simulink model "example_3_cascaded_attitude"  (R2016a)
settings: Solver=VariableStepAuto  StartTime=0.0  StopTime=Tsim  MaxStep=0.01  RelTol=1e-3
values from neighbouring files (symbols this model uses):
  ref_A = [4, 4, 4]    [init.m]
  ref_b = [0, 0, 0]    [init.m]
  ref_p = [1, 2, 3]    [init.m]
  ref_w = [0,0,0]    [init.m]
libraries: aerolibtransform2 x5, vrlib x3
settings Model: Creator=mgreiff  LastModifiedBy=mgreiff

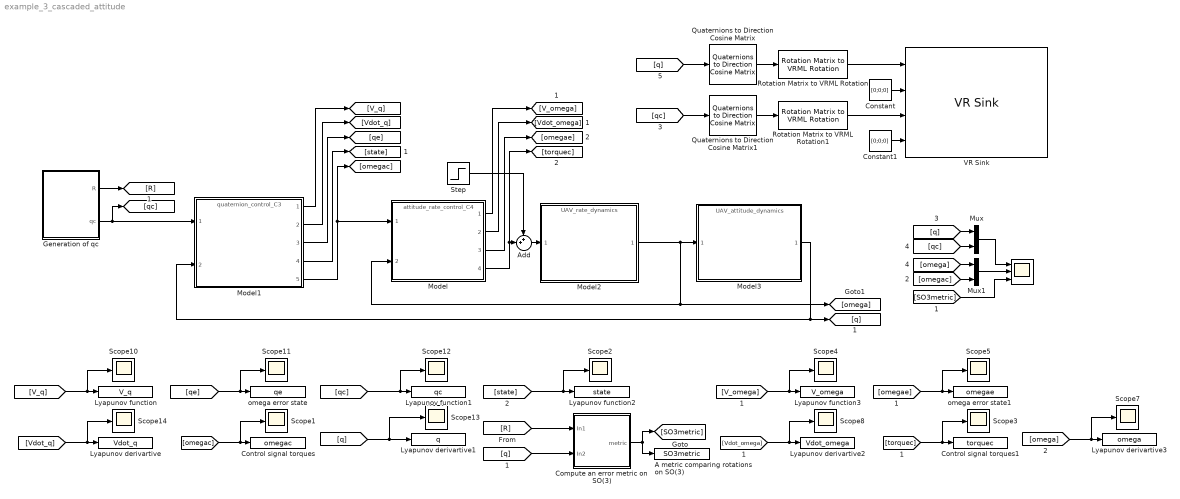
== system example_3_cascaded_attitude ==
  "                                     " : Scope  NumInputPorts=3
  A metric comparing rotations on SO(3) : ToWorkspace  VariableName=SO3metric  SaveFormat=Timeseries  SampleTime=-1
  Add : Sum  Inputs=++|
  Compute an error metric on SO(3) : Subsystem
  Constant : Constant  Value=[0;0;0]
  Constant1 : Constant  Value=[0;0;0]
  Control signal torques : ToWorkspace  VariableName=omegac  SaveFormat=Timeseries  SampleTime=-1
  Control signal torques1 : ToWorkspace  VariableName=torquec  SaveFormat=Timeseries  SampleTime=-1
  Generation of qc : Subsystem
  Lyapunov derivartive : ToWorkspace  VariableName=Vdot_q  SaveFormat=Timeseries  SampleTime=-1
  Lyapunov derivartive1 : ToWorkspace  VariableName=q  SaveFormat=Timeseries  SampleTime=-1
  Lyapunov derivartive2 : ToWorkspace  VariableName=Vdot_omega  SaveFormat=Timeseries  SampleTime=-1
  Lyapunov derivartive3 : ToWorkspace  VariableName=omega  SaveFormat=Timeseries  SampleTime=-1
  Lyapunov function : ToWorkspace  VariableName=V_q  SaveFormat=Timeseries  SampleTime=-1
  Lyapunov function1 : ToWorkspace  VariableName=qc  SaveFormat=Timeseries  SampleTime=-1
  Lyapunov function2 : ToWorkspace  VariableName=state  SaveFormat=Timeseries  SampleTime=-1
  Lyapunov function3 : ToWorkspace  VariableName=V_omega  SaveFormat=Timeseries  SampleTime=-1
  Model : ModelReference  ModelNameDialog=attitude_rate_control_C4.slx  SimulationMode=Normal  ModelReferenceVersion=1.37
  Model1 : ModelReference  ModelNameDialog=quaternion_control_C3.slx  SimulationMode=Normal  ModelReferenceVersion=1.25
  Model2 : ModelReference  ModelNameDialog=UAV_rate_dynamics.slx  SimulationMode=Normal  ModelReferenceVersion=1.9
  Model3 : ModelReference  ModelNameDialog=UAV_attitude_dynamics.slx  SimulationMode=Normal  ModelReferenceVersion=1.15
  Mux : Mux  Inputs=2
  Mux1 : Mux  Inputs=2
  Quaternions to Direction Cosine Matrix : aerolibtransform2/Quaternions to  Direction Cosine Matrix
  Quaternions to Direction Cosine Matrix1 : aerolibtransform2/Quaternions to  Direction Cosine Matrix
  Rotation Matrix to VRML Rotation : vrlib/Utilities/Rotation Matrix to VRML Rotation  maxzero=1e-12
  Rotation Matrix to VRML Rotation1 : vrlib/Utilities/Rotation Matrix to VRML Rotation  maxzero=1e-12
  Scope{1..5,7..8,10..14} (12 alike) : Scope
  Step : Step  Time=5  After=0  SampleTime=0
  VR Sink : vrlib/VR Sink  InstantiateOnLoad=on  SampleTime=-1  ViewEnable=on  RemoteChange=off  RemoteView=off  FieldsWritten=body_axis.rotation.4.1.1.double#body_axis.translation.3.1.1.double#reference_axis.rotation.4.1.1.double#reference_axis.translation.3.1.1.double  WorldFileName=my_coordinate_systems.wrl  AutoView=on  VideoDimensions=[]  AllowVariableSize=off
  omega error state : ToWorkspace  VariableName=qe  SaveFormat=Timeseries  SampleTime=-1
  omega error state1 : ToWorkspace  VariableName=omegae  SaveFormat=Timeseries  SampleTime=-1
  wires:
  [V_q] -> Lyapunov function/1, Scope10/1
  [Vdot_q] -> Lyapunov derivartive/1, Scope14/1
  [qc] -> Lyapunov function1/1, Scope12/1
  [q] -> Lyapunov derivartive1/1, Scope13/1
  [qe] -> omega error state/1, Scope11/1
  Model1/1 -> [V_q]
  Model1/2 -> [Vdot_q]
  Model1/3 -> [qe]
  [omegac] -> Control signal torques/1, Scope1/1
  Generation of qc/1(R) -> [R]
  [R] -> Compute an error metric on SO(3)/1(In1)
  [q] -> Compute an error metric on SO(3)/2(In2)
  Compute an error metric on SO(3)/1(metric) -> A metric comparing rotations on SO(3)/1, [SO3metric]
  [state] -> Lyapunov function2/1, Scope2/1
  Model1/4 -> [state]
  Model/4 -> Add/2, [torquec]
  Model2/1 -> Model/2, [omega], Model3/1
  Model3/1 -> Model1/2, [q]
  Model/1 -> [V_omega]
  Model/2 -> [Vdot_omega]
  Model/3 -> [omegae]
  [V_omega] -> Lyapunov function3/1, Scope4/1
  [Vdot_omega] -> Lyapunov derivartive2/1, Scope8/1
  [omega] -> Lyapunov derivartive3/1, Scope7/1
  [omegae] -> omega error state1/1, Scope5/1
  [torquec] -> Control signal torques1/1, Scope3/1
  [SO3metric] -> "                                     "/3
  Mux/1 -> "                                     "/1
  Mux1/1 -> "                                     "/2
  [qc] -> Mux/2
  [q] -> Mux/1
  [omega] -> Mux1/1
  [omegac] -> Mux1/2
  Rotation Matrix to VRML Rotation/1 -> VR Sink/1
  Quaternions to Direction Cosine Matrix/1 -> Rotation Matrix to VRML Rotation/1
  Rotation Matrix to VRML Rotation1/1 -> VR Sink/3
  Quaternions to Direction Cosine Matrix1/1 -> Rotation Matrix to VRML Rotation1/1
  [qc] -> Quaternions to Direction Cosine Matrix1/1
  [q] -> Quaternions to Direction Cosine Matrix/1
  Constant/1 -> VR Sink/2
  Constant1/1 -> VR Sink/4
  Model1/5 -> Model/1, [omegac]
  Step/1 -> Add/1
  Add/1 -> Model2/1
  Generation of qc/2("qc ") -> [qc], Model1/1

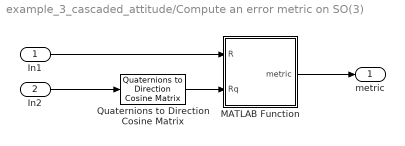
== system example_3_cascaded_attitude/Compute an error metric on SO(3) ==
  In1 : Inport
  In2 : Inport  Port=2
  MATLAB Function : MATLAB Function  TreatAsAtomicUnit=on
  Quaternions to Direction Cosine Matrix : aerolibtransform2/Quaternions to  Direction Cosine Matrix
  metric : Outport
  wires:
  MATLAB Function/1(metric) -> metric/1
  Quaternions to Direction Cosine Matrix/1 -> MATLAB Function/2(Rq)
  In1/1 -> MATLAB Function/1(R)
  In2/1 -> Quaternions to Direction Cosine Matrix/1

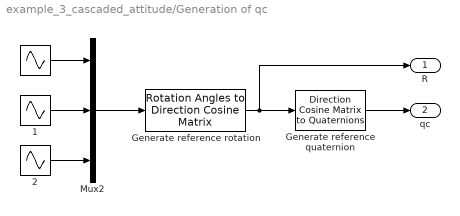
== system example_3_cascaded_attitude/Generation of qc ==
  " " : Sin  Amplitude=ref_A(1)  Bias=ref_b(1)  Frequency=ref_w(1)  Phase=ref_p(1)
  " 1" : Sin  Amplitude=ref_A(2)  Bias=ref_b(2)  Frequency=ref_w(2)  Phase=ref_p(2)
  " 2" : Sin  Amplitude=ref_A(3)  Bias=ref_b(3)  Frequency=ref_w(3)  Phase=ref_p(3)
  Generate reference quaternion : aerolibtransform2/Direction Cosine Matrix  to Quaternions
  Generate reference rotation : aerolibtransform2/Rotation Angles to Direction Cosine Matrix  rotationOrder=ZYX
  Mux2 : Mux  Inputs=3
  R : Outport
  "qc " : Outport  Port=2
  wires:
  " 1"/1 -> Mux2/2
  " "/1 -> Mux2/1
  " 2"/1 -> Mux2/3
  Generate reference rotation/1 -> Generate reference quaternion/1, R/1
  Generate reference quaternion/1 -> "qc "/1
  Mux2/1 -> Generate reference rotation/1

== matlab function example_3_cascaded_attitude/Compute an error metric on SO(3)/MATLAB Function ==
  data: R input; metric output; Rq input
function metric = fcn(R, Rq)
%#codegen
metric = trace(eye(3) - Rq'*R);
end
